simulink model "manual_acc_sim"  (R2022b)
settings: Solver=ode4  StartTime=0.0  StopTime=inf  FixedStep=Tc  RelTol=1e-3
values from neighbouring files (symbols this model uses):
  Kd = 1    [paraset.m]
  Ki = 2    [paraset.m]
  Kp = 10    [paraset.m]
  tau = 0.5    [paraset.m]
  Vx_d = 30    [paraset.m]
  Vx_i = 15    [paraset.m]
settings Model: Creator=user  LastModifiedBy=user
settings DataIOCC: ReturnWorkspaceOutputs=off

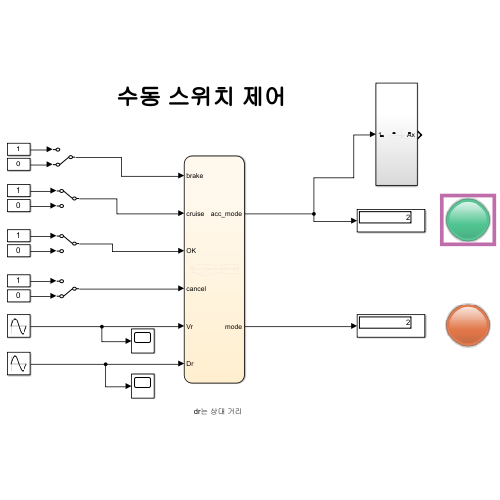
[thumbnail: Simulink's stored preview of the top-level diagram]
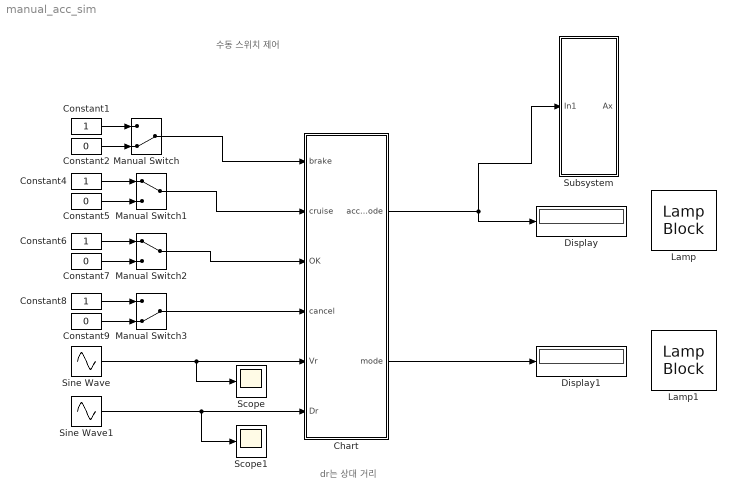
== system manual_acc_sim ==
  note: dr는 상대 거리
  note: 수동 스위치 제어
  Chart : Stateflow chart  TreatAsAtomicUnit=on
  Constant{1,4,6,8} (4 alike) : Constant
  Constant{2,5,7,9} (4 alike) : Constant  Value=0
  Display : Display
  Display1 : Display
  Lamp : LampBlock  LabelPosition=Hide
  Lamp1 : LampBlock  LabelPosition=Hide
  Manual Switch : ManualSwitch  CurrentSetting=0
  Manual Switch1 : ManualSwitch
  Manual Switch2 : ManualSwitch
  Manual Switch3 : ManualSwitch  CurrentSetting=0
  Scope : Scope
  Scope1 : Scope
  Sine Wave : Sin  SampleTime=0
  Sine Wave1 : Sin  Amplitude=50  Bias=250  Frequency=0.1  SampleTime=0
  Subsystem : Subsystem
  wires:
  Chart/1(acc_mode) -> Display/1, Subsystem/1(In1)
  Constant1/1 -> Manual Switch/1
  Constant2/1 -> Manual Switch/2
  Constant4/1 -> Manual Switch1/1
  Constant5/1 -> Manual Switch1/2
  Constant6/1 -> Manual Switch2/1
  Constant7/1 -> Manual Switch2/2
  Constant8/1 -> Manual Switch3/1
  Constant9/1 -> Manual Switch3/2
  Manual Switch/1 -> Chart/1(brake)
  Manual Switch1/1 -> Chart/2(cruise)
  Manual Switch2/1 -> Chart/3(OK)
  Manual Switch3/1 -> Chart/4(cancel)
  Chart/2(mode) -> Display1/1
  Sine Wave/1 -> Scope/1, Chart/5(Vr)
  Sine Wave1/1 -> Scope1/1, Chart/6(Dr)

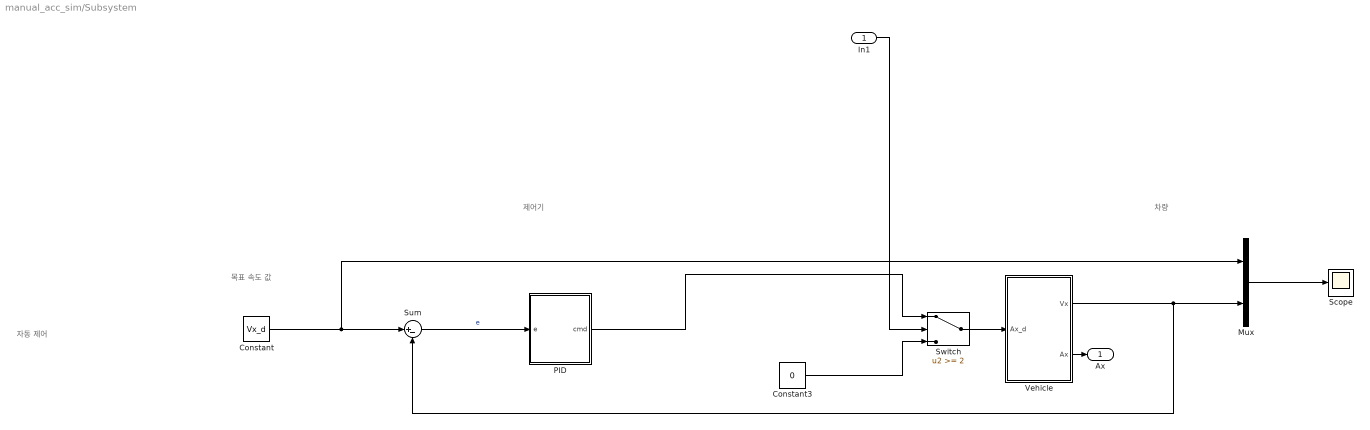
== system manual_acc_sim/Subsystem ==
  note: 목표 속도 값
  note: 차량
  note: 제어기
  note: 자동 제어
  In1 : Inport
  Constant : Constant  Value=Vx_d
  Constant3 : Constant  Value=0
  Mux : Mux  Inputs=2
  PID : Subsystem
  Scope : Scope
  Sum : Sum  Inputs=|+-
  Switch : Switch  Threshold=2  SaturateOnIntegerOverflow=off  InputSameDT=off
  Vehicle : Subsystem
  Ax : Outport
  wires:
  PID/1(cmd) -> Switch/1
  Mux/1 -> Scope/1
  Constant/1 -> Mux/1, Sum/1
  Sum/1 -> PID/1(e)  "e"
  Constant3/1 -> Switch/3
  Vehicle/1(Vx) -> Sum/2, Mux/2
  Switch/1 -> Vehicle/1(Ax_d)
  In1/1 -> Switch/2
  Vehicle/2(Ax) -> Ax/1

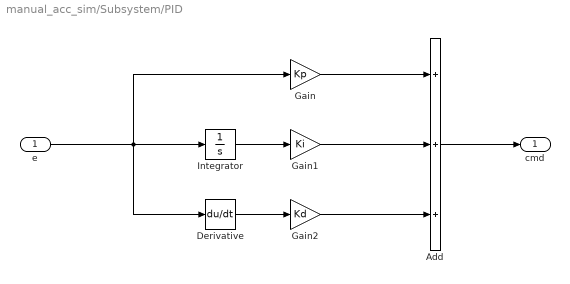
== system manual_acc_sim/Subsystem/PID ==
  e : Inport
  Add : Sum  Inputs=+++
  Derivative : Derivative
  Gain : Gain  Gain=Kp
  Gain1 : Gain  Gain=Ki
  Gain2 : Gain  Gain=Kd
  Integrator : Integrator
  cmd : Outport
  wires:
  Add/1 -> cmd/1
  e/1 -> Derivative/1, Integrator/1, Gain/1
  Gain/1 -> Add/1
  Gain1/1 -> Add/2
  Integrator/1 -> Gain1/1
  Derivative/1 -> Gain2/1
  Gain2/1 -> Add/3

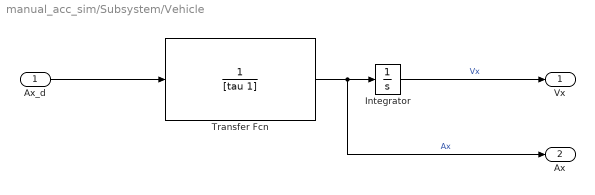
== system manual_acc_sim/Subsystem/Vehicle ==
  Ax_d : Inport
  Integrator : Integrator  InitialCondition=Vx_i
  Transfer Fcn : TransferFcn  Denominator=[tau 1]
  Vx : Outport
  Ax : Outport  Port=2
  wires:
  Transfer Fcn/1 -> Ax/1, Integrator/1  "Ax"
  Ax_d/1 -> Transfer Fcn/1
  Integrator/1 -> Vx/1  "Vx"

== stateflow chart manual_acc_sim/Chart ==
  state ACC_active
    acc_mode = 2;
    note: constant time gap
    state CC
      mode = 1;
    state CTG
      mode = 2;
    note: Vr = 앞차 거리 속도? Dr은 거리 차이 인가
    (default) -> CC
    CC -> CTG : [Vr < 0 & Dr <250]
    CTG -> CC : [Vr >= 0 | Dr > 250 ]
  state ACC_off
    acc_mode = 0;
  state ACC_standby
    acc_mode = 1;
  ACC_active -> ACC_off [order 3] : [cruise == 0]
  (default) -> ACC_off
  ACC_off -> ACC_standby : [cruise == 1 & brake == 0]
  ACC_standby -> ACC_active [order 1] : [OK == 1 & brake == 0]
  ACC_active -> ACC_standby [order 1] : [cancel == 1]
  ACC_standby -> ACC_off [order 2] : [cruise == 0]
  ACC_active -> ACC_off [order 2] : [brake == 1]
  ACC_standby -> ACC_off [order 3] : [brake == 1]
  data: brake input; cruise input; OK input; cancel input; acc_mode output; Vr input; Dr input; mode output
